simulink model "AutocarSim"  (R2014b)
settings: Solver=ode45  StartTime=0.0  StopTime=60  RelTol=1e-3
libraries: simulink x1
settings Model: Creator=think  LastModifiedBy=think

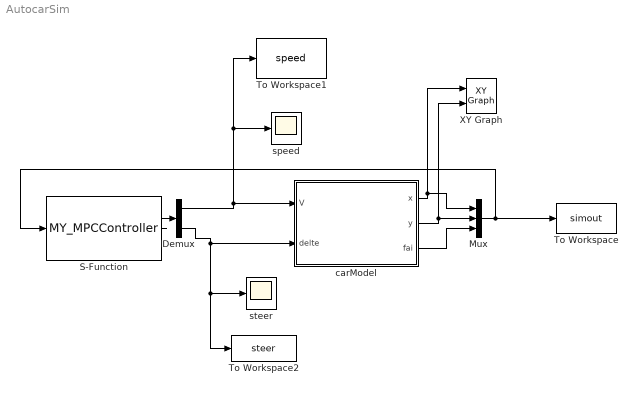
== system AutocarSim ==
  Demux : Demux  Outputs=2
  Mux : Mux  Inputs=3
  S-Function : S-Function  FunctionName=MY_MPCController  EnableBusSupport=off
  To Workspace : ToWorkspace  VariableName=simout  SaveFormat=Timeseries  SampleTime=-1
  To Workspace1 : ToWorkspace  VariableName=speed  SaveFormat=Timeseries  SampleTime=-1
  To Workspace2 : ToWorkspace  VariableName=steer  SaveFormat=Timeseries  SampleTime=-1
  XY Graph : simulink/Sinks/XY Graph  xmin=-100  xmax=100  ymin=-100  ymax=100  st=-1
  carModel : Subsystem
  speed : Scope
      settings: YMin=5.04  YMax=5.2
  steer : Scope
      settings: YMin=0.1  YMax=0.45
  wires:
  Demux/1 -> To Workspace1/1, speed/1, carModel/1(V)
  carModel/1(x) -> XY Graph/1, Mux/1
  carModel/2(y) -> XY Graph/2, Mux/2
  carModel/3(fai) -> Mux/3
  S-Function/1 -> Demux/1
  Mux/1 -> To Workspace/1, S-Function/1
  Demux/2 -> To Workspace2/1, steer/1, carModel/2(delte)

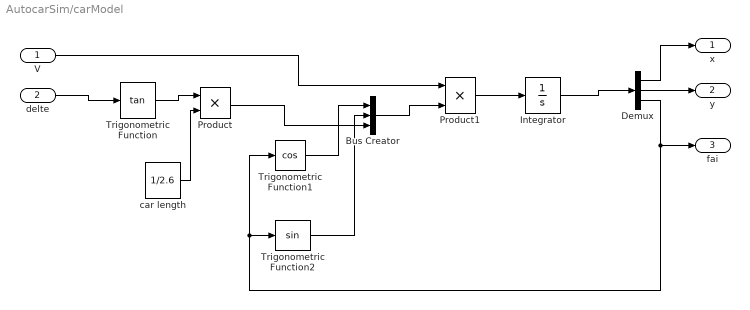
== system AutocarSim/carModel ==
  V : Inport
  delte : Inport  Port=2
  Bus Creator : BusCreator  Inputs=3
  Demux : Demux  Outputs=3
  Integrator : Integrator
  Product : Product
  Product1 : Product
  Trigonometric Function : Trigonometry  Operator=tan
  Trigonometric Function1 : Trigonometry  Operator=cos
  Trigonometric Function2 : Trigonometry
  car length : Constant  Value=1/2.6
  x : Outport
  y : Outport  Port=2
  fai : Outport  Port=3
  wires:
  delte/1 -> Trigonometric Function/1
  Bus Creator/1 -> Product1/2
  Product1/1 -> Integrator/1
  Demux/2 -> y/1
  Demux/3 -> Trigonometric Function1/1, Trigonometric Function2/1, fai/1
  car length/1 -> Product/2
  Trigonometric Function/1 -> Product/1
  Demux/1 -> x/1
  Integrator/1 -> Demux/1
  Trigonometric Function1/1 -> Bus Creator/1
  Trigonometric Function2/1 -> Bus Creator/2
  Product/1 -> Bus Creator/3
  V/1 -> Product1/1
